simulink model "Exp4"  (R2025b)
settings: Solver=VariableStepAuto  StartTime=0.0  StopTime=10000  RelTol=1e-3
libraries: dspstat3 x2, dspsrcs4 x2
settings Model: Creator=pc  LastModifiedBy=pc

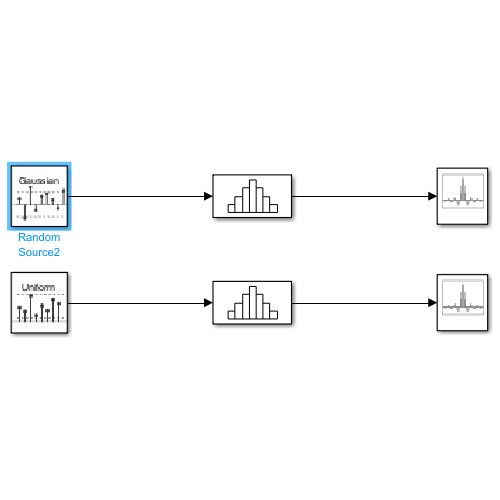
[thumbnail: Simulink's stored preview of the top-level diagram]
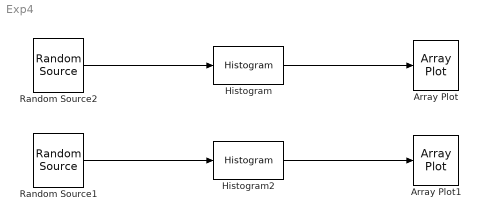
== system Exp4 ==
  Array Plot : ArrayPlot  WindowPosition=[283.000000,134.000000,800.000000,500.000000,]  ScopeFrameLocation=window  YLimits=[-0.16100346040238764 0.31632653959761214]
  Array Plot1 : ArrayPlot  WindowPosition=[283.000000,134.000000,800.000000,500.000000,]  ScopeFrameLocation=window  YLimits=[-0.43018711162065104 1.9579848751483415]
  Histogram : dspstat3/Histogram  umin=-5  umax=5  nbins=50  operateOver=Entire input  Dimension=1  normalized=on  run=on  reset=on  trigtype=None  colComp=on  roundingMode=Floor  overflowMode=off  accumDataTypeStr=Inherit: Same as product output  accumLastDataTypeStr=Inherit: Same as product output
  Histogram2 : dspstat3/Histogram  umin=-5  umax=5  nbins=50  operateOver=Entire input  Dimension=1  normalized=on  run=on  reset=on  trigtype=None  colComp=on  roundingMode=Floor  overflowMode=off  accumDataTypeStr=Inherit: Same as product output  accumLastDataTypeStr=Inherit: Same as product output
  Random Source1 : dspsrcs4/Random Source  SrcType=Uniform  MinVal=0  MaxVal=1  MeanVal=0  VarVal=1  RepMode=Not repeatable  rawSeed=1  IsInherit=off  SampTime=1/1000  SampFrame=1  OutComplex=Real  DataType=double  SimulateUsing=Interpreted execution
  Random Source2 : dspsrcs4/Random Source  SrcType=Gaussian  MinVal=0  MaxVal=1  MeanVal=0  VarVal=1  RepMode=Not repeatable  rawSeed=1  IsInherit=off  SampTime=1/1000  SampFrame=1  OutComplex=Real  DataType=double  SimulateUsing=Interpreted execution
  wires:
  Histogram2/1 -> Array Plot1/1
  Histogram/1 -> Array Plot/1
  Random Source2/1 -> Histogram/1
  Random Source1/1 -> Histogram2/1
